simulink model "Quad_Plant_top"  (R2023b)
settings: Solver=FixedStepAuto  StartTime=0.0  StopTime=inf  RelTol=1e-3
undefined symbols (not defined in the file): Payload, SampleTime
libraries: uavmavlinklib x6
settings Model: Creator=The MathWorks, Inc.  LastModifiedBy=The MathWorks, Inc.
settings SolverCC: AlgebraicLoopSolver=TrustRegion
settings OptimizationCC: ReuseModelBlockBuffer=off
settings DebuggingCC: UnconnectedInputMsg=warning  UnconnectedOutputMsg=warning  UnconnectedLineMsg=warning
settings ModelReferenceCC: EnableRefExpFcnMdlSchedulingChecks=on
settings RTWCC: DLArmComputeVersion=19.05

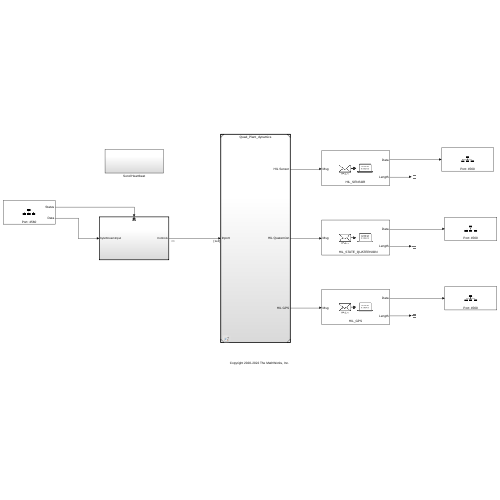
[thumbnail: Simulink's stored preview of the top-level diagram]
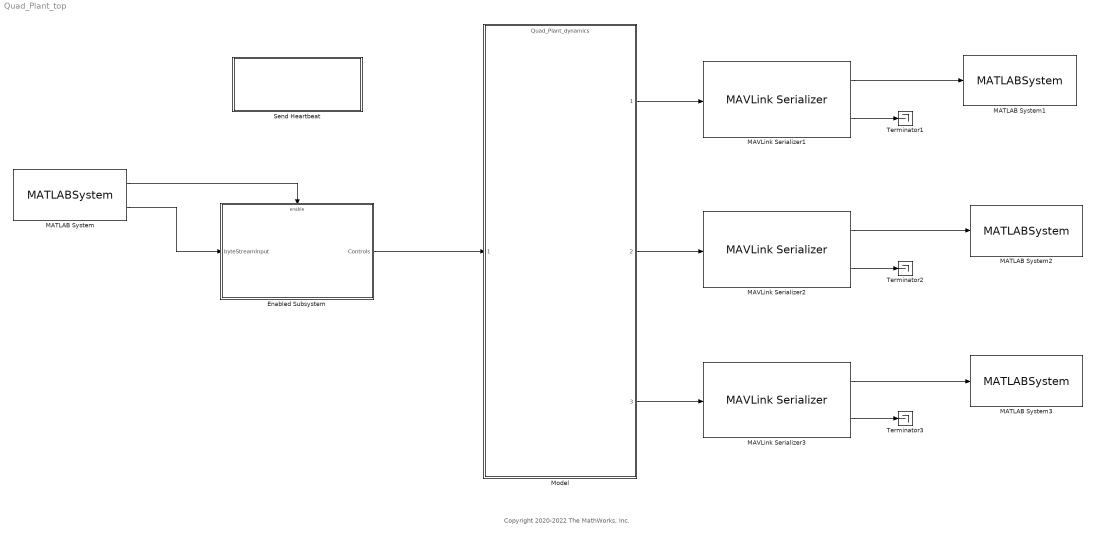
== system Quad_Plant_top ==
  note: Copyright 2020-2022 The MathWorks, Inc.
  Enabled Subsystem : Subsystem  TreatAsAtomicUnit=on
  MATLAB System : MATLABSystem  System=px4HostTarget_TCPIP_Read  Length=50  SampleTime=SampleTime
      mask Type: px4HostTarget_TCPIP_Read
      mask Display:
      | color('white');
      | plot([100,100,100,100]*1,[100,100,100,100]*1);
      | plot([100,100,100,100]*0,[100,100,100,100]*0);
      | color('black');
      | sppkgroot = strrep(codertarget.pixhawk.internal.getSpPkgRootDir(),'\','/');
      | image(fullfile(sppkgroot,'resources','TCP.jpg'),'center')
      | color('black');
      | text(50,12,sprintf('Port: %d',4560) ,'horizontalAlignment', 'center');
      | port_label('output',1,'Status');
      | port_label('output',2,'Data');
  MATLAB System1 : MATLABSystem  System=px4HostTarget_TCPIP_Write
      mask Type: px4HostTarget_TCPIP_Write
      mask Display:
      | color('white');
      | plot([100,100,100,100]*1,[100,100,100,100]*1);
      | plot([100,100,100,100]*0,[100,100,100,100]*0);
      | color('black');
      | sppkgroot = strrep(codertarget.pixhawk.internal.getSpPkgRootDir(),'\','/');
      | image(fullfile(sppkgroot,'resources','TCP.jpg'),'center')
      | color('black');
      | text(50,12,sprintf('Port: %d',4560) ,'horizontalAlignment', 'center');
  MATLAB System2 : MATLABSystem  System=px4HostTarget_TCPIP_Write
      mask Type: px4HostTarget_TCPIP_Write
      mask Display:
      | color('white');
      | plot([100,100,100,100]*1,[100,100,100,100]*1);
      | plot([100,100,100,100]*0,[100,100,100,100]*0);
      | color('black');
      | sppkgroot = strrep(codertarget.pixhawk.internal.getSpPkgRootDir(),'\','/');
      | image(fullfile(sppkgroot,'resources','TCP.jpg'),'center')
      | color('black');
      | text(50,12,sprintf('Port: %d',4560) ,'horizontalAlignment', 'center');
  MATLAB System3 : MATLABSystem  System=px4HostTarget_TCPIP_Write
      mask Type: px4HostTarget_TCPIP_Write
      mask Display:
      | color('white');
      | plot([100,100,100,100]*1,[100,100,100,100]*1);
      | plot([100,100,100,100]*0,[100,100,100,100]*0);
      | color('black');
      | sppkgroot = strrep(codertarget.pixhawk.internal.getSpPkgRootDir(),'\','/');
      | image(fullfile(sppkgroot,'resources','TCP.jpg'),'center')
      | color('black');
      | text(50,12,sprintf('Port: %d',4560) ,'horizontalAlignment', 'center');
  MAVLink Serializer1 : uavmavlinklib/MAVLink Serializer  dialectSource=Select from standard MAVLink dialects  dialect=common.xml  dialectCustom=common.xml  version=2  messageType=HIL_SENSOR
  MAVLink Serializer2 : uavmavlinklib/MAVLink Serializer  dialectSource=Select from standard MAVLink dialects  dialect=common.xml  dialectCustom=common.xml  version=2  messageType=HIL_STATE_QUATERNION
  MAVLink Serializer3 : uavmavlinklib/MAVLink Serializer  dialectSource=Select from standard MAVLink dialects  dialect=common.xml  dialectCustom=common.xml  version=2  messageType=HIL_GPS
  Model : ModelReference  ModelNameDialog=Quad_Plant_dynamics.slx  SimulationMode=Normal  ModelReferenceVersion=7.1
  Send Heartbeat : Subsystem
  Terminator1 : Terminator
  Terminator2 : Terminator
  Terminator3 : Terminator
  wires:
  Enabled Subsystem/1(Controls) -> Model/1
  Model/1 -> MAVLink Serializer1/1
  MAVLink Serializer1/1 -> MATLAB System1/1
  Model/2 -> MAVLink Serializer2/1
  MAVLink Serializer2/1 -> MATLAB System2/1
  Model/3 -> MAVLink Serializer3/1
  MAVLink Serializer1/2 -> Terminator1/1
  MAVLink Serializer2/2 -> Terminator2/1
  MAVLink Serializer3/2 -> Terminator3/1
  MAVLink Serializer3/1 -> MATLAB System3/1
  MATLAB System/2 -> Enabled Subsystem/1(byteStreamInput)
  MATLAB System/1 -> Enabled Subsystem/Enable

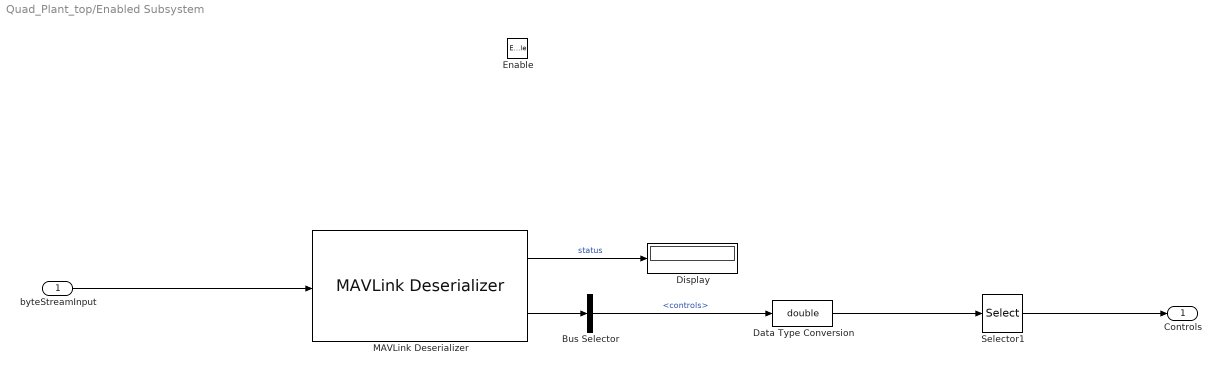
== system Quad_Plant_top/Enabled Subsystem ==
  byteStreamInput : Inport
  Enable : EnablePort
  Bus Selector : BusSelector  OutputSignals=Payload.controls
  Data Type Conversion : DataTypeConversion  OutDataTypeStr=double  SaturateOnIntegerOverflow=off  RndMeth=Floor
  Display : Display
  MAVLink Deserializer : uavmavlinklib/MAVLink Deserializer  dialectSource=Select from standard MAVLink dialects  dialect=common.xml  dialectCustom=common.xml  version=2  messageType=HIL_ACTUATOR_CONTROLS  inputDataLength=off  SystemIDFilter=off  systemID=1  ComponentIDFilter=off  componentID=1  queueMsg=off  queueMsgSize=50  dropNum=off
  Selector1 : Selector  InputPortWidth=16  IndexOptions=Index vector (dialog)  Indices=[1:4]  OutputSizes=1
  Controls : Outport
  wires:
  byteStreamInput/1 -> MAVLink Deserializer/1
  MAVLink Deserializer/2 -> Bus Selector/1
  Bus Selector/1 -> Data Type Conversion/1  "<controls>"
  MAVLink Deserializer/1 -> Display/1  "status"
  Data Type Conversion/1 -> Selector1/1
  Selector1/1 -> Controls/1

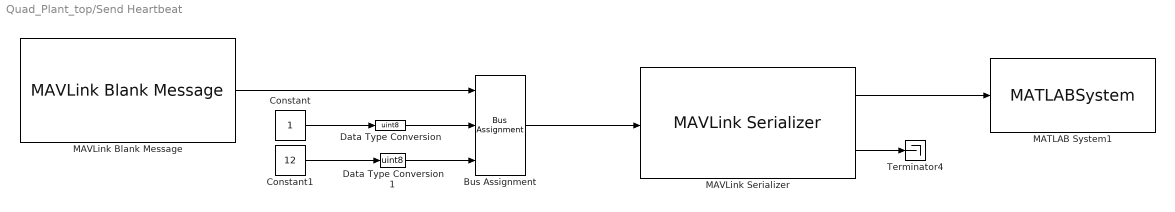
== system Quad_Plant_top/Send Heartbeat ==
  Bus Assignment : BusAssignment  AssignedSignals=Payload.autopilot,Payload.type
  Constant : Constant  SampleTime=SampleTime
  Constant1 : Constant  Value=12  SampleTime=SampleTime
  Data Type Conversion : DataTypeConversion  OutDataTypeStr=uint8  SaturateOnIntegerOverflow=off  RndMeth=Floor
  Data Type Conversion1 : DataTypeConversion  OutDataTypeStr=uint8  SaturateOnIntegerOverflow=off  RndMeth=Floor
  MATLAB System1 : MATLABSystem  System=px4HostTarget_TCPIP_Write
      mask Type: px4HostTarget_TCPIP_Write
      mask Display:
      | color('white');
      | plot([100,100,100,100]*1,[100,100,100,100]*1);
      | plot([100,100,100,100]*0,[100,100,100,100]*0);
      | color('black');
      | sppkgroot = strrep(codertarget.pixhawk.internal.getSpPkgRootDir(),'\','/');
      | image(fullfile(sppkgroot,'resources','TCP.jpg'),'center')
      | color('black');
      | text(50,12,sprintf('Port: %d',4560) ,'horizontalAlignment', 'center');
  MAVLink Blank Message : uavmavlinklib/MAVLink Blank Message  dialectSource=Select from standard MAVLink dialects  dialect=common.xml  dialectCustom=common.xml  version=2  messageType=HEARTBEAT  SystemID=2  ComponentID=51  SampleTime=SampleTime
  MAVLink Serializer : uavmavlinklib/MAVLink Serializer  dialectSource=Select from standard MAVLink dialects  dialect=common.xml  dialectCustom=common.xml  version=2  messageType=HEARTBEAT
  Terminator4 : Terminator
  wires:
  Bus Assignment/1 -> MAVLink Serializer/1
  Constant/1 -> Data Type Conversion/1
  MAVLink Serializer/1 -> MATLAB System1/1
  Data Type Conversion1/1 -> Bus Assignment/3
  Data Type Conversion/1 -> Bus Assignment/2
  MAVLink Serializer/2 -> Terminator4/1
  Constant1/1 -> Data Type Conversion1/1
  MAVLink Blank Message/1 -> Bus Assignment/1
